simulink model "leon_chen_TDPBehaviourSim2"  (R2020b)
settings: Solver=FixedStepDiscrete  StartTime=0.0  StopTime=inf  RelTol=1e-3  EnableMultiTasking=on
values from neighbouring files (symbols this model uses):
  angThresh = pi/16    (= 0.196349540849)    [GameParameters.m]
  attackerKickSpeed = 0.3    [GameParameters.m]
  AwayFormation1 = [9.5 4 pi ... (first row only)    [FormationPoses.m]    (also in GameParameters.m)
  ballThresh = playerRadius + 0.03    (= 0.11)    [GameParameters.m]
  distThresh = 0.1    [GameParameters.m]
  fieldCenter = [mean(fieldLimitsX) mean(fieldLimitsY)]    [GameParameters.m]
  fieldLimitsX = [1 10]    [GameParameters.m]
  fieldLimitsY = [1 7]    [GameParameters.m]
  goalPosts = [1  2.7 2 ... (first row only)    [GameParameters.m]
  HomeFormation1 = [1.5 4 0 ... (first row only)    [FormationPoses.m]    (also in GameParameters.m)
  maxSpeed = 0.1    [GameParameters.m]
  maxTurnSpeed = 0.05    [GameParameters.m]
  playerRadius = 0.08    [GameParameters.m]
  robotDetectorAngle = 0    [GameParameters.m]
  robotDetectorFOV = 4.15    [GameParameters.m]
  robotDetectorMaxHits = 7    [GameParameters.m]
  robotDetectorOffset = [0 0]    [GameParameters.m]
  robotDetectorRange = 10    [GameParameters.m]
  sampleTime = 0.5    [GameParameters.m]
undefined symbols (not defined in the file or in its folder): DiscIntNeverNeededParam
libraries: mobileRoboticsLib x28, soccerRobotLib x16
(part 1 of 2)
settings Model: Creator=2683935i  LastModifiedBy=2692920R
settings SolverCC: AutoInsertRateTranBlk=on
settings DataIOCC: SaveOutput=off  SaveTime=off
settings OptimizationCC: DefaultParameterBehavior=Inlined  InlineInvariantSignals=on  EnhancedBackFolding=on  PassReuseOutputArgsAs=Individual arguments  StateBitsets=on  DataBitsets=on  ZeroExternalMemoryAtStartup=off  ZeroInternalMemoryAtStartup=off  NoFixptDivByZeroProtection=on  LifeSpan=1  OptimizeBlockOrder=speed  DifferentSizesBufferReuse=on  EfficientTunableParamExpr=on
settings DebuggingCC: MultiTaskRateTransMsg=warning  ParameterTunabilityLossMsg=error
settings HardwareCC: ProdBitPerPointer=32  ProdBitPerSizeT=32  ProdBitPerPtrDiffT=32  ProdLargestAtomicFloat=None  ProdIntDivRoundTo=Floor  ProdWordSize=32  ProdHWDeviceType=Generic->Custom
settings SFSimCC: MATLABDynamicMemAlloc=off
settings RTWCC: Description=Embedded Coder  SystemTargetFile=ert.tlc  TLCOptions=-p0  GenCodeOnly=on  TemplateMakefile=ert_default_tmf  GenerateReport=on  RTWVerbose=off  IncludeHyperlinkInReport=on  LaunchReport=on
settings CodeAppCC: ForceParamTrailComments=on  IgnoreCustomStorageClasses=off  OperatorAnnotations=on  SimulinkDataObjDesc=on  SFDataObjDesc=on  CustomSymbolStrGlobalVar=rt$N$M  CustomSymbolStrType=$N$M  CustomSymbolStrFcn=$N$M$F  CustomSymbolStrMacro=$N$M  InsertBlockDesc=on
settings ERTTargetCC: TargetLangStandard=C99 (ISO)  GenerateSampleERTMain=on  IncludeMdlTerminateFcn=off  SuppressErrorStatus=on  SupportAbsoluteTime=off  PurelyIntegerCode=on  SupportNonFinite=off  SupportComplex=off  InlinedParameterPlacement=NonHierarchical  RootIOFormat=Structure reference  ERTCustomFileTemplate=example_file_process.tlc

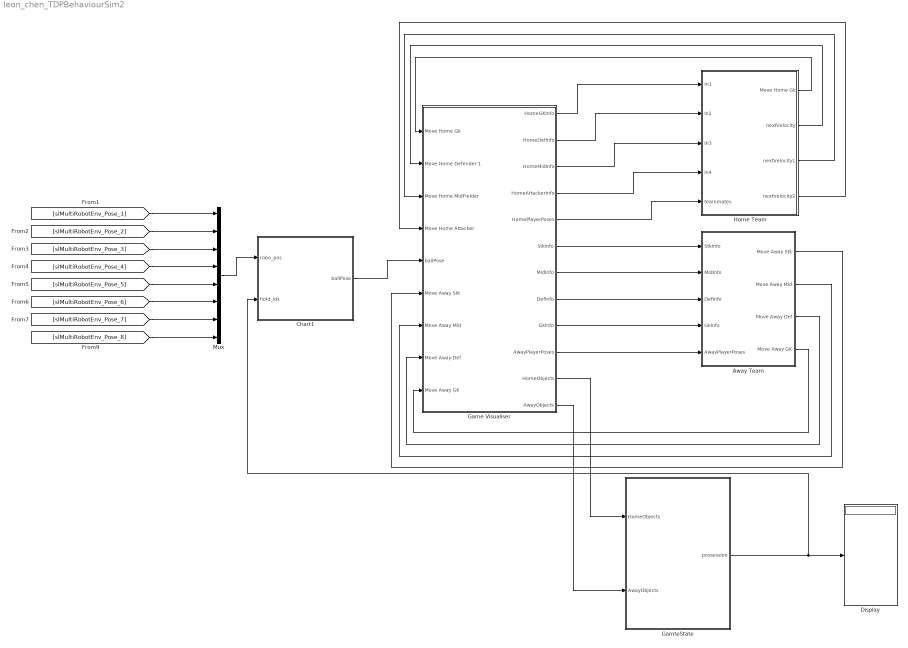
== system leon_chen_TDPBehaviourSim2 ==
  Away Team : Subsystem
  Chart1 : Stateflow chart  TreatAsAtomicUnit=on
  Display : Display
  Game Visualiser : Subsystem
  GamteState : Stateflow chart  TreatAsAtomicUnit=on
  Home Team : Subsystem
  Mux : Mux  Inputs=8
  wires:
  Away Team/2(Move Away Mid) -> Game Visualiser/7(Move Away Mid)
  Home Team/4(nextVelocity2) -> Game Visualiser/4(Move Home Attacker)
  Game Visualiser/5(HomePlayerPoses) -> Home Team/5(teammates)
  Home Team/1(Move Home Gk) -> Game Visualiser/1(Move Home Gk)
  Game Visualiser/1(HomeGKInfo) -> Home Team/1(In1)
  Home Team/2(nextVelocity) -> Game Visualiser/2(Move Home Defender 1)
  Away Team/4(Move Away GK) -> Game Visualiser/9(Move Away GK)
  Home Team/3(nextVelocity1) -> Game Visualiser/3(Move Home MidFielder)
  Game Visualiser/7(MidInfo) -> Away Team/2(MidInfo)
  Away Team/3(Move Away Def) -> Game Visualiser/8(Move Away Def)
  Chart1/1(ballPose) -> Game Visualiser/5(ballPose)
  Game Visualiser/9(GkInfo) -> Away Team/4(GkInfo)
  Game Visualiser/8(DefInfo) -> Away Team/3(DefInfo)
  Game Visualiser/6(StkInfo) -> Away Team/1(StkInfo)
  Game Visualiser/3(HomeMidInfo) -> Home Team/3(In3)
  Game Visualiser/4(HomeAttackerInfo) -> Home Team/4(In4)
  Game Visualiser/2(HomeDefInfo) -> Home Team/2(In2)
  Away Team/1(Move Away Stk) -> Game Visualiser/6(Move Away Stk)
  Game Visualiser/10(AwayPlayerPoses) -> Away Team/5(AwayPlayerPoses)
  GamteState/1(possession) -> Chart1/2(hold_idx), Display/1
  Game Visualiser/11(HomeObjects) -> GamteState/1(HomeObjects)
  Game Visualiser/12(AwayObjects) -> GamteState/2(AwayObjects)
  [slMultiRobotEnv_Pose_1] -> Mux/1
  [slMultiRobotEnv_Pose_2] -> Mux/2
  [slMultiRobotEnv_Pose_3] -> Mux/3
  [slMultiRobotEnv_Pose_4] -> Mux/4
  [slMultiRobotEnv_Pose_5] -> Mux/5
  [slMultiRobotEnv_Pose_6] -> Mux/6
  [slMultiRobotEnv_Pose_7] -> Mux/7
  [slMultiRobotEnv_Pose_8] -> Mux/8
  Mux/1 -> Chart1/1(robo_pos)

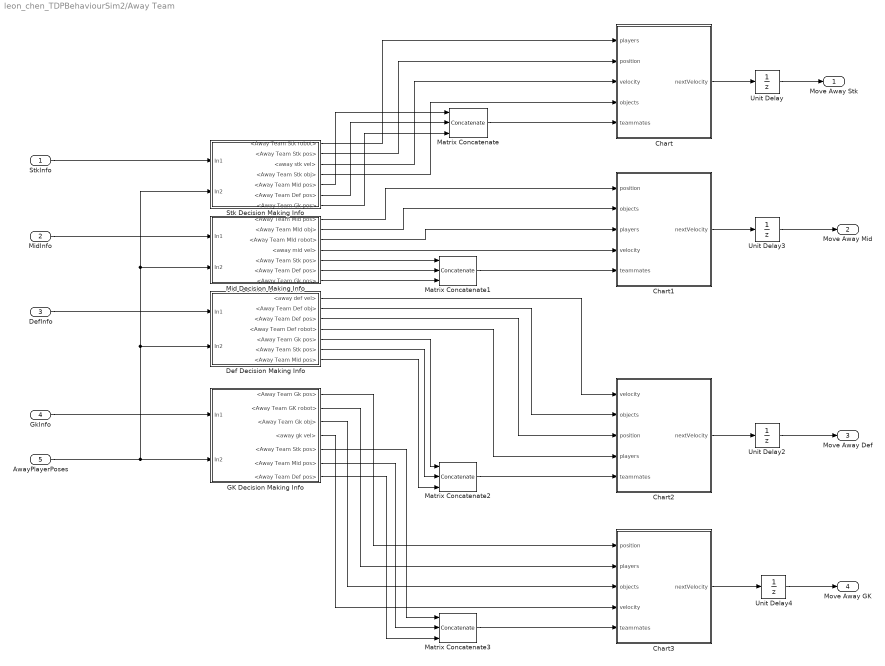
== system leon_chen_TDPBehaviourSim2/Away Team ==
  StkInfo : Inport
  MidInfo : Inport  Port=2
  DefInfo : Inport  Port=3
  GkInfo : Inport  Port=4
  AwayPlayerPoses : Inport  Port=5
  Chart : Stateflow chart  TreatAsAtomicUnit=on
      settings: PortSchema="{\"entries\":[{\"content\":{\"sides\":[{\"content\":{\"connectorIds\":[\"In3\",\"In1\",\"In2\",\"In5\",\"In4\"]},\"type\":\"ConnectorPlacement.EquallySpacedRectSide\",\"uuid\":\"cf890ef0-0ec1-422c-ab9c-1628c873ebf0\"},{\"content\":{\"connectorIds\":[\"Out1\"],\"side\":\"RIGHT\"},\"type\":\"ConnectorPlacement.EquallySpacedRectSide\",\"uuid\":\"0000e457-9393-40de-9950-8ff794b83dda\"},{\"content\":{\"connectorIds\":[],\"side\":\"TOP\"},\"type\":\"ConnectorPlacement.EquallySpacedRectSide\",\"uuid\":\"7dd8e30a-3952-4d7c-b255-0e0c48dee19a\"}]},\"type\":\"ConnectorPlacement.EquallySpacedConnector\",\"uuid\":\"e8168788-1535-41f0-a84f-110f92e839bd\"}],\"packageUris\":[\"http://schema.mathworks.com/mf0/Connector/R2020b\"],\"version\":\"1.0\"}"
  Chart1 : Stateflow chart  TreatAsAtomicUnit=on
      settings: PortSchema="{\"entries\":[{\"content\":{\"sides\":[{\"content\":{\"connectorIds\":[\"In1\",\"In5\",\"In3\",\"In2\",\"In4\"]},\"type\":\"ConnectorPlacement.EquallySpacedRectSide\",\"uuid\":\"cf890ef0-0ec1-422c-ab9c-1628c873ebf0\"},{\"content\":{\"connectorIds\":[\"Out1\"],\"side\":\"RIGHT\"},\"type\":\"ConnectorPlacement.EquallySpacedRectSide\",\"uuid\":\"0000e457-9393-40de-9950-8ff794b83dda\"},{\"content\":{\"connectorIds\":[],\"side\":\"TOP\"},\"type\":\"ConnectorPlacement.EquallySpacedRectSide\",\"uuid\":\"7dd8e30a-3952-4d7c-b255-0e0c48dee19a\"}]},\"type\":\"ConnectorPlacement.EquallySpacedConnector\",\"uuid\":\"e8168788-1535-41f0-a84f-110f92e839bd\"}],\"packageUris\":[\"http://schema.mathworks.com/mf0/Connector/R2020b\"],\"version\":\"1.0\"}"
  Chart2 : Stateflow chart  TreatAsAtomicUnit=on
      settings: PortSchema="{\"entries\":[{\"content\":{\"sides\":[{\"content\":{\"connectorIds\":[\"In2\",\"In5\",\"In1\",\"In3\",\"In4\"]},\"type\":\"ConnectorPlacement.EquallySpacedRectSide\",\"uuid\":\"cf890ef0-0ec1-422c-ab9c-1628c873ebf0\"},{\"content\":{\"connectorIds\":[\"Out1\"],\"side\":\"RIGHT\"},\"type\":\"ConnectorPlacement.EquallySpacedRectSide\",\"uuid\":\"0000e457-9393-40de-9950-8ff794b83dda\"},{\"content\":{\"connectorIds\":[],\"side\":\"TOP\"},\"type\":\"ConnectorPlacement.EquallySpacedRectSide\",\"uuid\":\"7dd8e30a-3952-4d7c-b255-0e0c48dee19a\"}]},\"type\":\"ConnectorPlacement.EquallySpacedConnector\",\"uuid\":\"e8168788-1535-41f0-a84f-110f92e839bd\"}],\"packageUris\":[\"http://schema.mathworks.com/mf0/Connector/R2020b\"],\"version\":\"1.0\"}"
  Chart3 : Stateflow chart  TreatAsAtomicUnit=on
      settings: PortSchema="{\"entries\":[{\"content\":{\"sides\":[{\"content\":{\"connectorIds\":[\"In1\",\"In3\",\"In5\",\"In2\",\"In4\"]},\"type\":\"ConnectorPlacement.EquallySpacedRectSide\",\"uuid\":\"cf890ef0-0ec1-422c-ab9c-1628c873ebf0\"},{\"content\":{\"connectorIds\":[\"Out1\"],\"side\":\"RIGHT\"},\"type\":\"ConnectorPlacement.EquallySpacedRectSide\",\"uuid\":\"0000e457-9393-40de-9950-8ff794b83dda\"},{\"content\":{\"connectorIds\":[],\"side\":\"TOP\"},\"type\":\"ConnectorPlacement.EquallySpacedRectSide\",\"uuid\":\"7dd8e30a-3952-4d7c-b255-0e0c48dee19a\"}]},\"type\":\"ConnectorPlacement.EquallySpacedConnector\",\"uuid\":\"e8168788-1535-41f0-a84f-110f92e839bd\"}],\"packageUris\":[\"http://schema.mathworks.com/mf0/Connector/R2020b\"],\"version\":\"1.0\"}"
  Def Decision Making Info : Subsystem
  GK Decision Making Info : Subsystem
  Matrix Concatenate{,1..3} (4 alike) : Concatenate  NumInputs=3  Mode=Multidimensional array
  Mid Decision Making Info : Subsystem
  Stk Decision Making Info : Subsystem
  Unit Delay{,2..4} (4 alike) : UnitDelay  SampleTime=-1  HasFrameUpgradeWarning=on
  Move Away Stk : Outport
  Move Away Mid : Outport  Port=2
  Move Away Def : Outport  Port=3
  Move Away GK : Outport  Port=4
  wires:
  Def Decision Making Info/7(<Away Team Mid pos>) -> Matrix Concatenate2/3
  Def Decision Making Info/6(<Away Team Stk pos>) -> Matrix Concatenate2/2
  AwayPlayerPoses/1 -> Stk Decision Making Info/2(In2), Mid Decision Making Info/2(In2), Def Decision Making Info/2(In2), GK Decision Making Info/2(In2)
  Def Decision Making Info/3(<Away Team Def pos>) -> Chart2/1(position)
  Matrix Concatenate3/1 -> Chart3/4(teammates)
  Unit Delay/1 -> Move Away Stk/1
  Stk Decision Making Info/6(<Away Team Def pos>) -> Matrix Concatenate/2
  Stk Decision Making Info/5(<Away Team Mid pos>) -> Matrix Concatenate/1
  Mid Decision Making Info/6(<Away Team Def pos>) -> Matrix Concatenate1/2
  Def Decision Making Info/1(<away def vel>) -> Chart2/2(velocity)
  Mid Decision Making Info/1(<Away Team Mid pos>) -> Chart1/1(position)
  Mid Decision Making Info/7(<Away Team Gk pos>) -> Matrix Concatenate1/3
  Mid Decision Making Info/4(<away mid vel>) -> Chart1/2(velocity)
  GK Decision Making Info/7(<Away Team Def pos>) -> Matrix Concatenate3/3
  GK Decision Making Info/2(<Away Team GK robot>) -> Chart3/3(players)
  GK Decision Making Info/1(<Away Team Gk pos>) -> Chart3/1(position)
  Matrix Concatenate/1 -> Chart/4(teammates)
  Stk Decision Making Info/4(<Away Team Stk obj>) -> Chart/5(objects)
  Chart1/1(nextVelocity) -> Unit Delay3/1
  Mid Decision Making Info/2(<Away Team MId obj>) -> Chart1/5(objects)
  Chart2/1(nextVelocity) -> Unit Delay2/1
  GkInfo/1 -> GK Decision Making Info/1(In1)
  Mid Decision Making Info/3(<Away Team MId robot>) -> Chart1/3(players)
  GK Decision Making Info/6(<Away Team Mid pos>) -> Matrix Concatenate3/2
  Chart/1(nextVelocity) -> Unit Delay/1
  Unit Delay4/1 -> Move Away GK/1
  Mid Decision Making Info/5(<Away Team Stk pos>) -> Matrix Concatenate1/1
  Def Decision Making Info/2(<Away Team Def obj>) -> Chart2/5(objects)
  Stk Decision Making Info/1(<Away Team Stk robot>) -> Chart/3(players)
  StkInfo/1 -> Stk Decision Making Info/1(In1)
  Def Decision Making Info/4(<Away Team Def robot>) -> Chart2/3(players)
  Chart3/1(nextVelocity) -> Unit Delay4/1
  Matrix Concatenate1/1 -> Chart1/4(teammates)
  GK Decision Making Info/3(<Away Team Gk obj>) -> Chart3/5(objects)
  Stk Decision Making Info/3(<away stk vel>) -> Chart/2(velocity)
  MidInfo/1 -> Mid Decision Making Info/1(In1)
  GK Decision Making Info/4(<away gk vel>) -> Chart3/2(velocity)
  Stk Decision Making Info/2(<Away Team Stk pos>) -> Chart/1(position)
  Matrix Concatenate2/1 -> Chart2/4(teammates)
  Stk Decision Making Info/7(<Away Team Gk pos>) -> Matrix Concatenate/3
  DefInfo/1 -> Def Decision Making Info/1(In1)
  Def Decision Making Info/5(<Away Team Gk pos>) -> Matrix Concatenate2/1
  Unit Delay2/1 -> Move Away Def/1
  GK Decision Making Info/5(<Away Team Stk pos>) -> Matrix Concatenate3/1
  Unit Delay3/1 -> Move Away Mid/1

== system leon_chen_TDPBehaviourSim2/Chart1/BallDynamics.InBounds.BallFree ==
  Action Port : ActionPort
      settings: CopyFcn=Stateflow.SLINSF.SimulinkMan.removeBlockPreDeleteFcn  PreDeleteFcn=Stateflow.SLINSF.SimulinkMan.unsafePredeleteFcn
  Gain : Gain  Gain=-0.25
  Position Integrator : DiscreteIntegrator  InitialCondition=fieldCenter  SampleTime=-1  StateName=ballPos  ICPrevOutput=DiscIntNeverNeededParam  ICPrevScaledInput=DiscIntNeverNeededParam
  Signal Specification : SignalSpecification  Dimensions=[1 2]
  Velocity Integrator : DiscreteIntegrator  InitialCondition=[0 0]  SampleTime=-1  StateName=ballVel  ICPrevOutput=DiscIntNeverNeededParam  ICPrevScaledInput=DiscIntNeverNeededParam
  ballPose : Outport  VectorParamsAs1DForOutWhenUnconnected=off
  wires:
  Gain/1 -> Velocity Integrator/1
  Velocity Integrator/1 -> Signal Specification/1
  Position Integrator/1 -> ballPose/1
  Signal Specification/1 -> Position Integrator/1, Gain/1

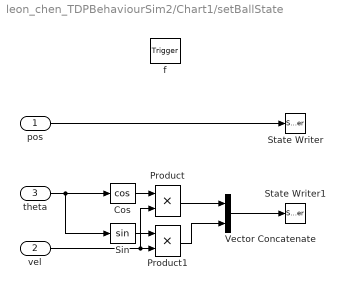
== system leon_chen_TDPBehaviourSim2/Chart1/setBallState ==
  pos : Inport  OutDataTypeStr=double  PortDimensions=[1 2]
  vel : Inport  Port=2  OutDataTypeStr=double  PortDimensions=1
  theta : Inport  Port=3  OutDataTypeStr=double  PortDimensions=1
  f : TriggerPort  TriggerType=function-call  VariantControl=(inherit)
      settings: CopyFcn=Stateflow.SLINSF.SimulinkMan.removeBlockPreDeleteFcn  PreDeleteFcn=Stateflow.SLINSF.SimulinkMan.unsafePredeleteFcn
  Cos : Trigonometry  Operator=cos
  Product : Product
  Product1 : Product
  Sin : Trigonometry
  State Writer : StateWriter  StateOwnerBlock=../../BallDynamics.InBounds.BallFree/Position Integrator  StateName=ballPos
  State Writer1 : StateWriter  StateOwnerBlock=../../BallDynamics.InBounds.BallFree/Velocity Integrator  StateName=ballVel
  Vector Concatenate : Concatenate  Mode=Multidimensional array  ConcatenateDimension=2
  wires:
  Vector Concatenate/1 -> State Writer1/1
  Product1/1 -> Vector Concatenate/2
  Product/1 -> Vector Concatenate/1
  theta/1 -> Cos/1, Sin/1
  Sin/1 -> Product1/1
  vel/1 -> Product1/2, Product/2
  Cos/1 -> Product/1
  pos/1 -> State Writer/1

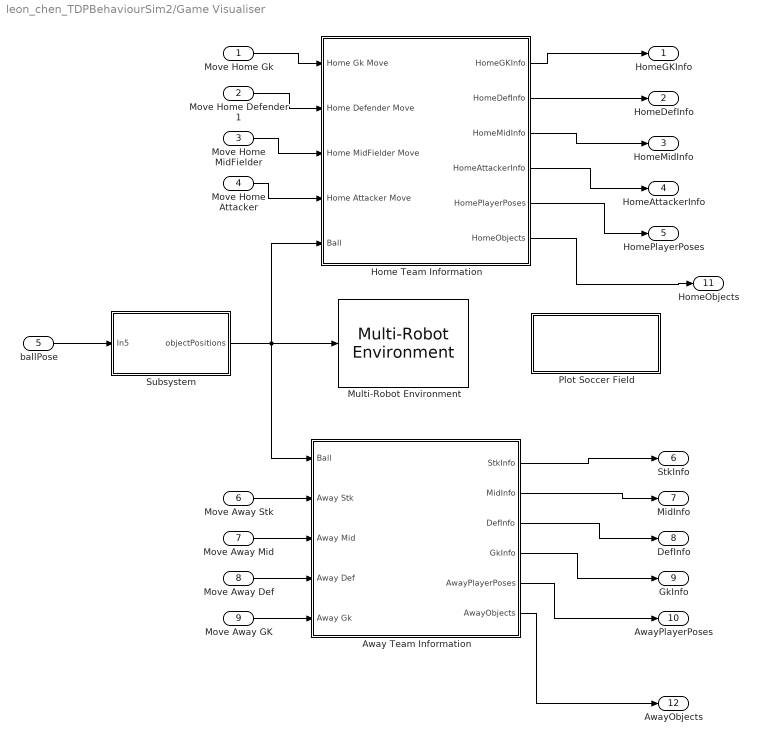
== system leon_chen_TDPBehaviourSim2/Game Visualiser ==
  Move Home Gk : Inport
  Move Home Defender 1 : Inport  Port=2
  Move Home MidFielder : Inport  Port=3
  Move Home Attacker : Inport  Port=4
  ballPose : Inport  Port=5
  Move Away Stk : Inport  Port=6
  Move Away Mid : Inport  Port=7
  Move Away Def : Inport  Port=8
  Move Away GK : Inport  Port=9
  Away Team Information : Subsystem
  Home Team Information : Subsystem
  Multi-Robot Environment : mobileRoboticsLib/Environments/Multi-Robot Environment  numRobots=numPlayers  mapName=map  showWaypoints=off  showObjects=on  objectColors=objColors  objectMarkers='o^^^^'  showRobotIds=on  plotSensorLines=off
      settings: SourceProductName=Mobile Robotics Simulation Toolbox
  Plot Soccer Field : MATLAB Function  TreatAsAtomicUnit=on
  Subsystem : Subsystem
  HomeGKInfo : Outport
  HomeDefInfo : Outport  Port=2
  HomeMidInfo : Outport  Port=3
  HomeAttackerInfo : Outport  Port=4
  HomePlayerPoses : Outport  Port=5
  StkInfo : Outport  Port=6
  MidInfo : Outport  Port=7
  DefInfo : Outport  Port=8
  GkInfo : Outport  Port=9
  AwayPlayerPoses : Outport  Port=10
  HomeObjects : Outport  Port=11
  AwayObjects : Outport  Port=12
  wires:
  Move Away Stk/1 -> Away Team Information/2(Away Stk)
  Move Home Defender 1/1 -> Home Team Information/2(Home Defender Move)
  Move Home MidFielder/1 -> Home Team Information/3(Home MidFielder Move)
  Move Away GK/1 -> Away Team Information/5("Away Gk ")
  Move Away Mid/1 -> Away Team Information/3(Away Mid)
  Move Away Def/1 -> Away Team Information/4(Away Def)
  Move Home Attacker/1 -> Home Team Information/4(Home Attacker Move)
  Move Home Gk/1 -> Home Team Information/1(Home Gk Move)
  Home Team Information/1(HomeGKInfo) -> HomeGKInfo/1
  Home Team Information/2(HomeDefInfo) -> HomeDefInfo/1
  Home Team Information/3(HomeMidInfo) -> HomeMidInfo/1
  Home Team Information/4(HomeAttackerInfo) -> HomeAttackerInfo/1
  Home Team Information/5(HomePlayerPoses) -> HomePlayerPoses/1
  Away Team Information/1(StkInfo) -> StkInfo/1
  Away Team Information/2(MidInfo) -> MidInfo/1
  Away Team Information/3(DefInfo) -> DefInfo/1
  Away Team Information/4(GkInfo) -> GkInfo/1
  Away Team Information/5(AwayPlayerPoses) -> AwayPlayerPoses/1
  Subsystem/1(objectPositions) -> Multi-Robot Environment/1, Away Team Information/1(Ball), Home Team Information/5(Ball)
  ballPose/1 -> Subsystem/1(In5)
  Home Team Information/6(HomeObjects) -> HomeObjects/1
  Away Team Information/6(AwayObjects) -> AwayObjects/1

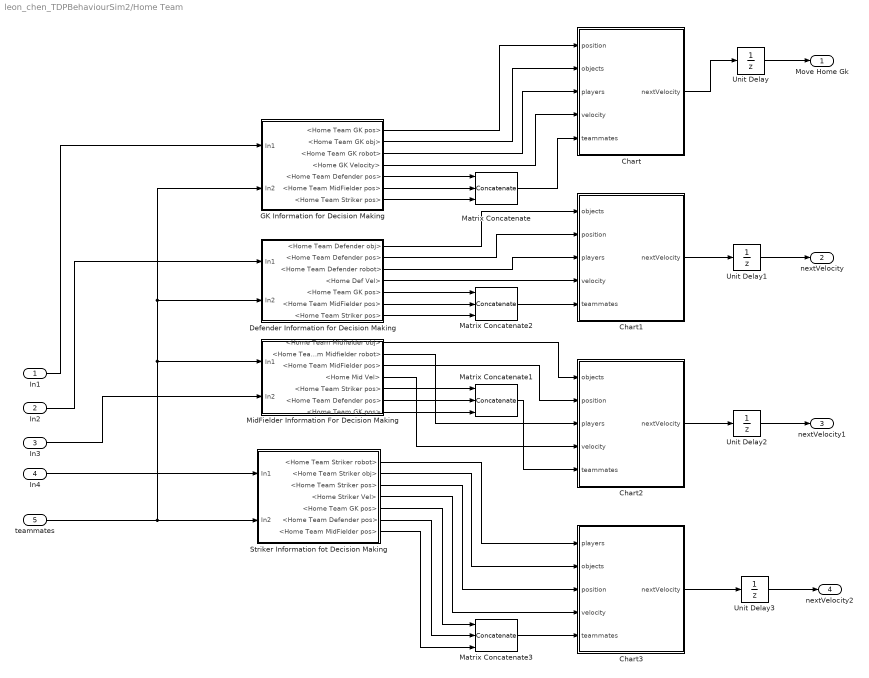
== system leon_chen_TDPBehaviourSim2/Home Team ==
  In1 : Inport
  In2 : Inport  Port=2
  In3 : Inport  Port=3
  In4 : Inport  Port=4
  teammates : Inport  Port=5
  Chart : Stateflow chart  TreatAsAtomicUnit=on
      settings: PortSchema="{\"entries\":[{\"content\":{\"sides\":[{\"content\":{\"connectorIds\":[\"In1\",\"In5\",\"In3\",\"In2\",\"In4\"]},\"type\":\"ConnectorPlacement.EquallySpacedRectSide\",\"uuid\":\"cf890ef0-0ec1-422c-ab9c-1628c873ebf0\"},{\"content\":{\"connectorIds\":[\"Out1\"],\"side\":\"RIGHT\"},\"type\":\"ConnectorPlacement.EquallySpacedRectSide\",\"uuid\":\"0000e457-9393-40de-9950-8ff794b83dda\"},{\"content\":{\"connectorIds\":[],\"side\":\"TOP\"},\"type\":\"ConnectorPlacement.EquallySpacedRectSide\",\"uuid\":\"7dd8e30a-3952-4d7c-b255-0e0c48dee19a\"}]},\"type\":\"ConnectorPlacement.EquallySpacedConnector\",\"uuid\":\"e8168788-1535-41f0-a84f-110f92e839bd\"}],\"packageUris\":[\"http://schema.mathworks.com/mf0/Connector/R2020b\"],\"version\":\"1.0\"}"
  Chart1 : Stateflow chart  TreatAsAtomicUnit=on
      settings: PortSchema="{\"entries\":[{\"content\":{\"sides\":[{\"content\":{\"connectorIds\":[\"In5\",\"In1\",\"In3\",\"In2\",\"In4\"]},\"type\":\"ConnectorPlacement.EquallySpacedRectSide\",\"uuid\":\"cf890ef0-0ec1-422c-ab9c-1628c873ebf0\"},{\"content\":{\"connectorIds\":[\"Out1\"],\"side\":\"RIGHT\"},\"type\":\"ConnectorPlacement.EquallySpacedRectSide\",\"uuid\":\"0000e457-9393-40de-9950-8ff794b83dda\"},{\"content\":{\"connectorIds\":[],\"side\":\"TOP\"},\"type\":\"ConnectorPlacement.EquallySpacedRectSide\",\"uuid\":\"7dd8e30a-3952-4d7c-b255-0e0c48dee19a\"}]},\"type\":\"ConnectorPlacement.EquallySpacedConnector\",\"uuid\":\"e8168788-1535-41f0-a84f-110f92e839bd\"}],\"packageUris\":[\"http://schema.mathworks.com/mf0/Connector/R2020b\"],\"version\":\"1.0\"}"
  Chart2 : Stateflow chart  TreatAsAtomicUnit=on
      settings: PortSchema="{\"entries\":[{\"content\":{\"sides\":[{\"content\":{\"connectorIds\":[\"In4\",\"In5\",\"In2\",\"In1\",\"In3\"]},\"type\":\"ConnectorPlacement.EquallySpacedRectSide\",\"uuid\":\"cf890ef0-0ec1-422c-ab9c-1628c873ebf0\"},{\"content\":{\"connectorIds\":[\"Out1\"],\"side\":\"RIGHT\"},\"type\":\"ConnectorPlacement.EquallySpacedRectSide\",\"uuid\":\"0000e457-9393-40de-9950-8ff794b83dda\"},{\"content\":{\"connectorIds\":[],\"side\":\"TOP\"},\"type\":\"ConnectorPlacement.EquallySpacedRectSide\",\"uuid\":\"7dd8e30a-3952-4d7c-b255-0e0c48dee19a\"}]},\"type\":\"ConnectorPlacement.EquallySpacedConnector\",\"uuid\":\"e8168788-1535-41f0-a84f-110f92e839bd\"}],\"packageUris\":[\"http://schema.mathworks.com/mf0/Connector/R2020b\"],\"version\":\"1.0\"}"
  Chart3 : Stateflow chart  TreatAsAtomicUnit=on
      settings: PortSchema="{\"entries\":[{\"content\":{\"sides\":[{\"content\":{\"connectorIds\":[\"In3\",\"In5\",\"In1\",\"In2\",\"In4\"]},\"type\":\"ConnectorPlacement.EquallySpacedRectSide\",\"uuid\":\"cf890ef0-0ec1-422c-ab9c-1628c873ebf0\"},{\"content\":{\"connectorIds\":[\"Out1\"],\"side\":\"RIGHT\"},\"type\":\"ConnectorPlacement.EquallySpacedRectSide\",\"uuid\":\"0000e457-9393-40de-9950-8ff794b83dda\"},{\"content\":{\"connectorIds\":[],\"side\":\"TOP\"},\"type\":\"ConnectorPlacement.EquallySpacedRectSide\",\"uuid\":\"7dd8e30a-3952-4d7c-b255-0e0c48dee19a\"}]},\"type\":\"ConnectorPlacement.EquallySpacedConnector\",\"uuid\":\"e8168788-1535-41f0-a84f-110f92e839bd\"}],\"packageUris\":[\"http://schema.mathworks.com/mf0/Connector/R2020b\"],\"version\":\"1.0\"}"
  "Defender Information for Decision Making " : Subsystem
  GK Information for Decision Making : Subsystem
  Matrix Concatenate : Concatenate  NumInputs=3  Mode=Multidimensional array  ConcatenateDimension=2
  Matrix Concatenate1 : Concatenate  NumInputs=3  Mode=Multidimensional array  ConcatenateDimension=2
  Matrix Concatenate2 : Concatenate  NumInputs=3  Mode=Multidimensional array  ConcatenateDimension=2
  Matrix Concatenate3 : Concatenate  NumInputs=3  Mode=Multidimensional array
  MidFielder Information For Decision Making : Subsystem
  Striker Information fot Decision Making : Subsystem
  Unit Delay{,1..3} (4 alike) : UnitDelay  SampleTime=-1  HasFrameUpgradeWarning=on
  Move Home Gk : Outport
  nextVelocity : Outport  Port=2
  nextVelocity1 : Outport  Port=3
  nextVelocity2 : Outport  Port=4
  wires:
  "Defender Information for Decision Making "/7(<Home Team Striker pos>) -> Matrix Concatenate2/3
  Matrix Concatenate3/1 -> Chart3/4(teammates)
  Matrix Concatenate1/1 -> Chart2/3(teammates)
  Striker Information fot Decision Making/7(<Home Team MidFielder pos>) -> Matrix Concatenate3/3
  Striker Information fot Decision Making/4(<Home Striker Vel>) -> Chart3/2(velocity)
  "Defender Information for Decision Making "/3(<Home Team Defender robot>) -> Chart1/3(players)
  GK Information for Decision Making/1(<Home Team GK pos>) -> Chart/1(position)
  In2/1 -> "Defender Information for Decision Making "/1(In1)
  GK Information for Decision Making/4(<Home GK Velocity>) -> Chart/2(velocity)
  teammates/1 -> GK Information for Decision Making/2(In2), "Defender Information for Decision Making "/2(In2), MidFielder Information For Decision Making/1(In1), Striker Information fot Decision Making/2(In2)
  Chart/1(nextVelocity) -> Unit Delay/1
  In4/1 -> Striker Information fot Decision Making/1(In1)
  "Defender Information for Decision Making "/6(<Home Team MidFielder pos>) -> Matrix Concatenate2/2
  GK Information for Decision Making/7(<Home Team Striker pos>) -> Matrix Concatenate/3
  In3/1 -> MidFielder Information For Decision Making/2(In2)
  MidFielder Information For Decision Making/3(<Home Team MidFielder pos>) -> Chart2/5(position)
  GK Information for Decision Making/3(<Home Team GK robot>) -> Chart/3(players)
  "Defender Information for Decision Making "/1(<Home Team Defender obj>) -> Chart1/5(objects)
  In1/1 -> GK Information for Decision Making/1(In1)
  "Defender Information for Decision Making "/4(<Home Def Vel>) -> Chart1/2(velocity)
  GK Information for Decision Making/5(<Home Team Defender pos>) -> Matrix Concatenate/1
  MidFielder Information For Decision Making/2(<Home Team Midfielder robot>) -> Chart2/2(players)
  GK Information for Decision Making/6(<Home Team MidFielder pos>) -> Matrix Concatenate/2
  Matrix Concatenate2/1 -> Chart1/4(teammates)
  Striker Information fot Decision Making/6(<Home Team Defender pos>) -> Matrix Concatenate3/2
  MidFielder Information For Decision Making/5(<Home Team Striker pos>) -> Matrix Concatenate1/1
  Striker Information fot Decision Making/3(<Home Team Striker pos>) -> Chart3/1(position)
  MidFielder Information For Decision Making/7(<Home Team GK pos>) -> Matrix Concatenate1/3
  GK Information for Decision Making/2(<Home Team GK obj>) -> Chart/5(objects)
  MidFielder Information For Decision Making/4(<Home Mid Vel>) -> Chart2/1(velocity)
  MidFielder Information For Decision Making/1(<Home Team Midfielder obj>) -> Chart2/4(objects)
  Striker Information fot Decision Making/2(<Home Team Striker obj>) -> Chart3/5(objects)
  Striker Information fot Decision Making/1(<Home Team Striker robot>) -> Chart3/3(players)
  Striker Information fot Decision Making/5(<Home Team GK pos>) -> Matrix Concatenate3/1
  Unit Delay/1 -> Move Home Gk/1
  MidFielder Information For Decision Making/6(<Home Team Defender pos>) -> Matrix Concatenate1/2
  "Defender Information for Decision Making "/2(<Home Team Defender pos>) -> Chart1/1(position)
  "Defender Information for Decision Making "/5(<Home Team GK pos>) -> Matrix Concatenate2/1
  Unit Delay3/1 -> nextVelocity2/1
  Chart3/1(nextVelocity) -> Unit Delay3/1
  Chart2/1(nextVelocity) -> Unit Delay2/1
  Unit Delay2/1 -> nextVelocity1/1
  Unit Delay1/1 -> nextVelocity/1
  Chart1/1(nextVelocity) -> Unit Delay1/1
  Matrix Concatenate/1 -> Chart/4(teammates)

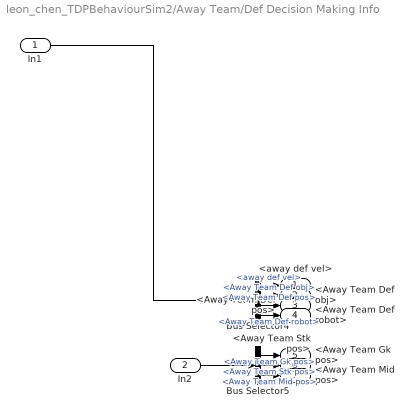
== system leon_chen_TDPBehaviourSim2/Away Team/Def Decision Making Info ==
  In1 : Inport
  In2 : Inport  Port=2
  Bus Selector4 : BusSelector  OutputSignals=away def vel,Away Team Def obj,Away Team Def pos,Away Team Def robot
  Bus Selector5 : BusSelector  OutputSignals=Away Team Gk pos,Away Team Stk pos,Away Team Mid pos
  <away def vel> : Outport
  <Away Team Def obj> : Outport  Port=2
  <Away Team Def pos> : Outport  Port=3
  <Away Team Def robot> : Outport  Port=4
  <Away Team Gk pos> : Outport  Port=5
  <Away Team Stk pos> : Outport  Port=6
  <Away Team Mid pos> : Outport  Port=7
  wires:
  Bus Selector5/2 -> <Away Team Stk pos>/1  "<Away Team Stk pos>"
  Bus Selector5/3 -> <Away Team Mid pos>/1  "<Away Team Mid pos>"
  Bus Selector4/2 -> <Away Team Def obj>/1  "<Away Team Def obj>"
  Bus Selector4/3 -> <Away Team Def pos>/1  "<Away Team Def pos>"
  Bus Selector4/1 -> <away def vel>/1  "<away def vel>"
  In2/1 -> Bus Selector5/1
  In1/1 -> Bus Selector4/1
  Bus Selector4/4 -> <Away Team Def robot>/1  "<Away Team Def robot>"
  Bus Selector5/1 -> <Away Team Gk pos>/1  "<Away Team Gk pos>"

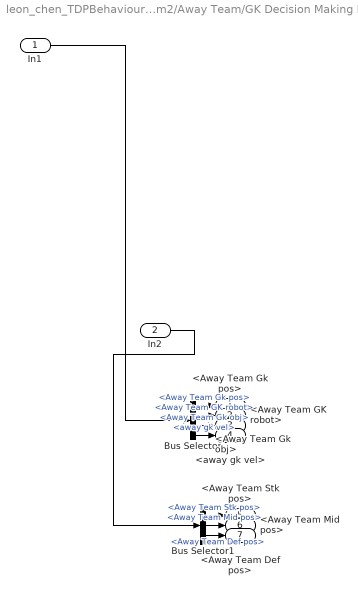
== system leon_chen_TDPBehaviourSim2/Away Team/GK Decision Making Info ==
  In1 : Inport
  In2 : Inport  Port=2
  Bus Selector : BusSelector  OutputSignals=Away Team Gk pos,Away Team GK robot,Away Team Gk obj,away gk vel
  Bus Selector1 : BusSelector  OutputSignals=Away Team Stk pos,Away Team Mid pos,Away Team Def pos
  <Away Team Gk pos> : Outport
  <Away Team GK robot> : Outport  Port=2
  <Away Team Gk obj> : Outport  Port=3
  <away gk vel> : Outport  Port=4
  <Away Team Stk pos> : Outport  Port=5
  <Away Team Mid pos> : Outport  Port=6
  <Away Team Def pos> : Outport  Port=7
  wires:
  In2/1 -> Bus Selector1/1
  Bus Selector/2 -> <Away Team GK robot>/1  "<Away Team GK robot>"
  Bus Selector/3 -> <Away Team Gk obj>/1  "<Away Team Gk obj>"
  In1/1 -> Bus Selector/1
  Bus Selector1/3 -> <Away Team Def pos>/1  "<Away Team Def pos>"
  Bus Selector/1 -> <Away Team Gk pos>/1  "<Away Team Gk pos>"
  Bus Selector1/1 -> <Away Team Stk pos>/1  "<Away Team Stk pos>"
  Bus Selector/4 -> <away gk vel>/1  "<away gk vel>"
  Bus Selector1/2 -> <Away Team Mid pos>/1  "<Away Team Mid pos>"

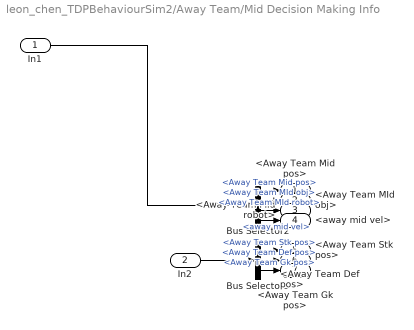
== system leon_chen_TDPBehaviourSim2/Away Team/Mid Decision Making Info ==
  In1 : Inport
  In2 : Inport  Port=2
  Bus Selector2 : BusSelector  OutputSignals=Away Team Mid pos,Away Team MId obj,Away Team MId robot,away mid vel
  Bus Selector3 : BusSelector  OutputSignals=Away Team Stk pos,Away Team Def pos,Away Team Gk pos
  <Away Team Mid pos> : Outport
  <Away Team MId obj> : Outport  Port=2
  <Away Team MId robot> : Outport  Port=3
  <away mid vel> : Outport  Port=4
  <Away Team Stk pos> : Outport  Port=5
  <Away Team Def pos> : Outport  Port=6
  <Away Team Gk pos> : Outport  Port=7
  wires:
  Bus Selector2/2 -> <Away Team MId obj>/1  "<Away Team MId obj>"
  Bus Selector3/1 -> <Away Team Stk pos>/1  "<Away Team Stk pos>"
  Bus Selector2/3 -> <Away Team MId robot>/1  "<Away Team MId robot>"
  In1/1 -> Bus Selector2/1
  Bus Selector3/2 -> <Away Team Def pos>/1  "<Away Team Def pos>"
  Bus Selector3/3 -> <Away Team Gk pos>/1  "<Away Team Gk pos>"
  In2/1 -> Bus Selector3/1
  Bus Selector2/1 -> <Away Team Mid pos>/1  "<Away Team Mid pos>"
  Bus Selector2/4 -> <away mid vel>/1  "<away mid vel>"

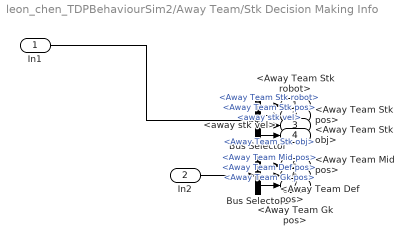
== system leon_chen_TDPBehaviourSim2/Away Team/Stk Decision Making Info ==
  In1 : Inport
  In2 : Inport  Port=2
  Bus Selector : BusSelector  OutputSignals=Away Team Stk robot,Away Team Stk pos,away stk vel,Away Team Stk obj
  Bus Selector1 : BusSelector  OutputSignals=Away Team Mid pos,Away Team Def pos,Away Team Gk pos
  <Away Team Stk robot> : Outport
  <Away Team Stk pos> : Outport  Port=2
  <away stk vel> : Outport  Port=3
  <Away Team Stk obj> : Outport  Port=4
  <Away Team Mid pos> : Outport  Port=5
  <Away Team Def pos> : Outport  Port=6
  <Away Team Gk pos> : Outport  Port=7
  wires:
  In2/1 -> Bus Selector1/1
  Bus Selector/3 -> <away stk vel>/1  "<away stk vel>"
  Bus Selector1/2 -> <Away Team Def pos>/1  "<Away Team Def pos>"
  Bus Selector/4 -> <Away Team Stk obj>/1  "<Away Team Stk obj>"
  Bus Selector1/3 -> <Away Team Gk pos>/1  "<Away Team Gk pos>"
  Bus Selector/1 -> <Away Team Stk robot>/1  "<Away Team Stk robot>"
  Bus Selector1/1 -> <Away Team Mid pos>/1  "<Away Team Mid pos>"
  Bus Selector/2 -> <Away Team Stk pos>/1  "<Away Team Stk pos>"
  In1/1 -> Bus Selector/1

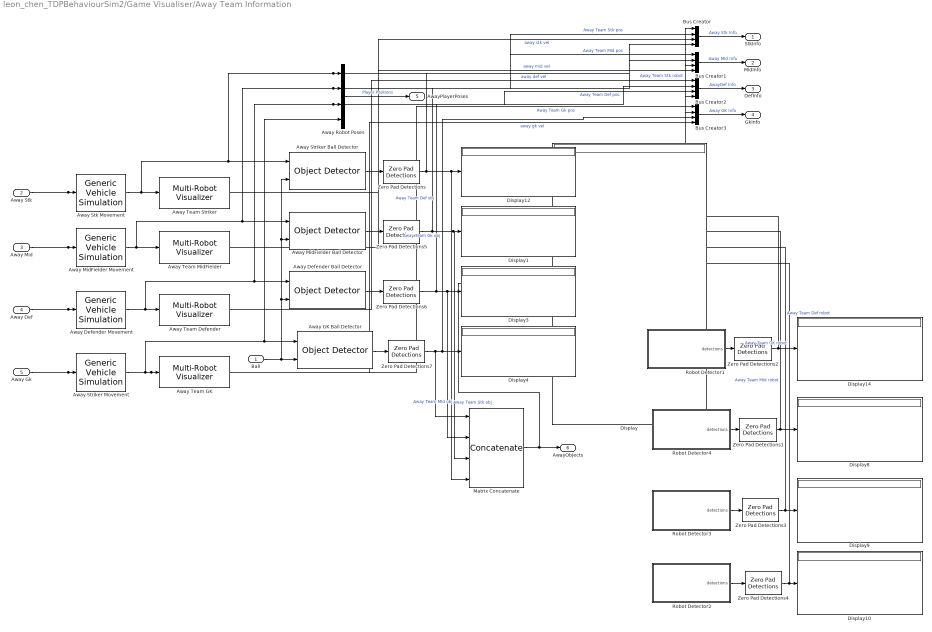
== system leon_chen_TDPBehaviourSim2/Game Visualiser/Away Team Information ==
  Ball : Inport
  Away Stk : Inport  Port=2
  Away Mid : Inport  Port=3
  Away Def : Inport  Port=4
  "Away Gk " : Inport  Port=5
  Away Defender Ball Detector : mobileRoboticsLib/Environments/Object Detector  mapName=map  sensorOffset=objDetectorOffset  sensorAngle=objDetectorAngle  fieldOfView=objDetectorFOV  maxRange=objDetectorRange  maxDetections=objDetectorMaxHits  sampleTime=sampleTime
      settings: SourceProductName=Mobile Robotics Simulation Toolbox
  Away Defender Movement : mobileRoboticsLib/Utilities/Generic Vehicle Simulation  initX=AwayFormation1(2,1)  initY=AwayFormation1(2,2)  initAngle=AwayFormation1(2,3)  Ts=0.05
      settings: SourceProductName=Mobile Robotics Simulation Toolbox
  Away GK Ball Detector : mobileRoboticsLib/Environments/Object Detector  mapName=map  sensorOffset=objDetectorOffset  sensorAngle=objDetectorAngle  fieldOfView=objDetectorFOV  maxRange=objDetectorRange  maxDetections=objDetectorMaxHits  sampleTime=sampleTime
      settings: SourceProductName=Mobile Robotics Simulation Toolbox
  Away MidFielder Ball Detector : mobileRoboticsLib/Environments/Object Detector  mapName=map  sensorOffset=objDetectorOffset  sensorAngle=objDetectorAngle  fieldOfView=objDetectorFOV  maxRange=objDetectorRange  maxDetections=objDetectorMaxHits  sampleTime=sampleTime
      settings: SourceProductName=Mobile Robotics Simulation Toolbox
  Away MidFielder Movement : mobileRoboticsLib/Utilities/Generic Vehicle Simulation  initX=AwayFormation1(3,1)  initY=AwayFormation1(3,2)  initAngle=AwayFormation1(3,3)  Ts=0.05
      settings: SourceProductName=Mobile Robotics Simulation Toolbox
  Away Robot Poses : BusCreator  Inputs=4
  Away Stk Movement : mobileRoboticsLib/Utilities/Generic Vehicle Simulation  initX=AwayFormation1(4,1)  initY=AwayFormation1(4,2)  initAngle=AwayFormation1(4,3)  Ts=0.05
      settings: SourceProductName=Mobile Robotics Simulation Toolbox
  Away Striker Ball Detector : mobileRoboticsLib/Environments/Object Detector  mapName=map  sensorOffset=objDetectorOffset  sensorAngle=objDetectorAngle  fieldOfView=objDetectorFOV  maxRange=objDetectorRange  maxDetections=objDetectorMaxHits  sampleTime=sampleTime
      settings: SourceProductName=Mobile Robotics Simulation Toolbox
  Away Striker Movement : mobileRoboticsLib/Utilities/Generic Vehicle Simulation  initX=AwayFormation1(1,1)  initY=AwayFormation1(1,2)  initAngle=AwayFormation1(1,3)  Ts=0.05
      settings: SourceProductName=Mobile Robotics Simulation Toolbox
  Away Team Defender : mobileRoboticsLib/Environments/Multi-Robot Visualizer  idx=7  radius=playerRadius  robotColor=awayTeamColor  showTraj=on  hasLidar=off  sensorOffset=[0,0]  scanAngles=[-pi/4 0 pi/4]  maxNumScans=0  hasObjDetector=on  objDetectorOffset=objDetectorOffset  objDetectorAngle=objDetectorAngle  objDetectorFOV=objDetectorFOV  objDetectorMaxRange=objDetectorRange  hasRobotDetector=on  robotDetectorOffset=robotDetectorOffset  robotDetectorAngle=robotDetectorAngle  robotDetectorFOV=robotDetectorFOV  robotDetectorMaxRange=robotDetectorMaxHits  robotDetectorNumDetections=0
      settings: SourceProductName=Mobile Robotics Simulation Toolbox
  Away Team GK : mobileRoboticsLib/Environments/Multi-Robot Visualizer  idx=8  radius=playerRadius  robotColor=awayGKColor  showTraj=on  hasLidar=off  sensorOffset=[0,0]  scanAngles=[-pi/4 0 pi/4]  maxNumScans=0  hasObjDetector=on  objDetectorOffset=objDetectorOffset  objDetectorAngle=objDetectorAngle  objDetectorFOV=objDetectorFOV  objDetectorMaxRange=objDetectorRange  hasRobotDetector=on  robotDetectorOffset=robotDetectorOffset  robotDetectorAngle=robotDetectorAngle  robotDetectorFOV=robotDetectorFOV  robotDetectorMaxRange=robotDetectorMaxHits  robotDetectorNumDetections=0
      settings: SourceProductName=Mobile Robotics Simulation Toolbox
  Away Team MidFielder : mobileRoboticsLib/Environments/Multi-Robot Visualizer  idx=6  radius=playerRadius  robotColor=awayTeamColor  showTraj=on  hasLidar=off  sensorOffset=[0,0]  scanAngles=[-pi/4 0 pi/4]  maxNumScans=0  hasObjDetector=on  objDetectorOffset=objDetectorOffset  objDetectorAngle=objDetectorAngle  objDetectorFOV=objDetectorFOV  objDetectorMaxRange=objDetectorRange  hasRobotDetector=on  robotDetectorOffset=robotDetectorOffset  robotDetectorAngle=robotDetectorAngle  robotDetectorFOV=robotDetectorFOV  robotDetectorMaxRange=robotDetectorMaxHits  robotDetectorNumDetections=0
      settings: SourceProductName=Mobile Robotics Simulation Toolbox
  Away Team Striker : mobileRoboticsLib/Environments/Multi-Robot Visualizer  idx=5  radius=playerRadius  robotColor=awayTeamColor  showTraj=on  hasLidar=off  sensorOffset=[0,0]  scanAngles=[-pi/4 0 pi/4]  maxNumScans=0  hasObjDetector=on  objDetectorOffset=objDetectorOffset  objDetectorAngle=objDetectorAngle  objDetectorFOV=objDetectorFOV  objDetectorMaxRange=objDetectorRange  hasRobotDetector=on  robotDetectorOffset=robotDetectorOffset  robotDetectorAngle=robotDetectorAngle  robotDetectorFOV=robotDetectorFOV  robotDetectorMaxRange=robotDetectorMaxHits  robotDetectorNumDetections=0
      settings: SourceProductName=Mobile Robotics Simulation Toolbox
  Bus Creator{,1..3} (4 alike) : BusCreator  Inputs=4
  Display{,1,3..4,8..10,12,14} (9 alike) : Display
  Matrix Concatenate : Concatenate  NumInputs=4  Mode=Multidimensional array
  Robot Detector1 : Subsystem  AncestorBlock=mobileRoboticsLib/Environments/Robot Detector  mask(Robot Detector){mapName=map, robotIdx=5, sensorOffset=robotDetectorOffset, sensorAngle=robotDetectorAngle, sensorFOV=robotDetectorFOV, maxRange=robotDetectorRange, maxDetections=robotDetectorMaxHits, sampleTime=sampleTime}
      mask prompts: mapName "Map Name"; robotIdx "Robot Index"; sensorOffset "Sensor offset (x,y) [m]"; sensorAngle "Sensor angle [rad]"; sensorFOV "Sensor field of view [rad]"; maxRange "Maximum range [rad]"; maxDetections "Maximum number of detections"; sampleTime "Sample Time"
      mask help: Robot Detector Simulator
      mask init:
      | % Find number of robots 
      | mrEnvBlks = find_system(bdroot,'FollowLinks','on','LookUnderMasks','on','MaskType','Multi-Robot Environment');
      | mrEnvBlk = mrEnvBlks{1};
      | if isempty(mrEnvBlk)
      |     error('No Multi-Robot Environment found in model.')
      | end
      | numRobots = evalin('base',get_param(mrEnvBlk,'numRobots'));
      | 
      | % Configure pose tags
      | poseSub = [gcb '/Poses'];
      | poseBlocks = find_system(poseSub,'FollowLinks','on','LookUnderMasks','on','BlockType','From');
      | for idx = 1:numel(poseBlocks)
      |     lh = get_param(poseBlocks{idx},'LineHandles');
      |     delete_line(lh.Outport);
      | end
      | delete_block(poseBlocks);
      | vecBlock = [poseSub '/Vector Concatenate'];
      | set_param(vecBlock,'NumInputs',num2str(numRobots));
      | for idx = 1:numRobots
      |     blkName = [poseSub '/From' num2str(idx)];
      |     blkPos = [0 30 200 50] + (idx-1)*[0 30 0 30];
      |     add_block('simulink/Signal Routing/From',blkName);
      |     set_param(blkName,'GotoTag',['slMultiRobotEnv_Pose_' num2str(idx)]);
      |     set_param(blkName,'Position',blkPos);
      |     add_line(poseSub,['From' num2str(idx) '/1'],['Vector Concatenate/' num2str(idx)]);
      | end
      mask Help: web('matlab: edit mrsDocRobotDetector')
      mask Callback mapName:
      | % Update the map in the Robot Detector system object inside the mask
      | mapName = get_param(gcb,'mapName');
      | blkName = [gcb '/Robot Detector'];
      | set_param(blkName,'mapName',mapName);
      mask Display:
      | idx = get_param(gcb,'robotIdx');
      | fprintf(['Robot ' idx '\n Detector'])
  Robot Detector2 : Subsystem  AncestorBlock=mobileRoboticsLib/Environments/Robot Detector  mask(Robot Detector){mapName=map, robotIdx=8, sensorOffset=robotDetectorOffset, sensorAngle=robotDetectorAngle, sensorFOV=robotDetectorFOV, maxRange=robotDetectorRange, maxDetections=robotDetectorMaxHits, sampleTime=sampleTime}
      mask prompts: mapName "Map Name"; robotIdx "Robot Index"; sensorOffset "Sensor offset (x,y) [m]"; sensorAngle "Sensor angle [rad]"; sensorFOV "Sensor field of view [rad]"; maxRange "Maximum range [rad]"; maxDetections "Maximum number of detections"; sampleTime "Sample Time"
      mask help: Robot Detector Simulator
      mask init: same as leon_chen_TDPBehaviourSim2/Game Visualiser/Away Team Information/Robot Detector1
      mask Help: web('matlab: edit mrsDocRobotDetector')
      mask Callback mapName:
      | % Update the map in the Robot Detector system object inside the mask
      | mapName = get_param(gcb,'mapName');
      | blkName = [gcb '/Robot Detector'];
      | set_param(blkName,'mapName',mapName);
      mask Display:
      | idx = get_param(gcb,'robotIdx');
      | fprintf(['Robot ' idx '\n Detector'])
  Robot Detector3 : Subsystem  AncestorBlock=mobileRoboticsLib/Environments/Robot Detector  mask(Robot Detector){mapName=map, robotIdx=7, sensorOffset=robotDetectorOffset, sensorAngle=robotDetectorAngle, sensorFOV=robotDetectorFOV, maxRange=robotDetectorRange, maxDetections=robotDetectorMaxHits, sampleTime=sampleTime}
      mask prompts: mapName "Map Name"; robotIdx "Robot Index"; sensorOffset "Sensor offset (x,y) [m]"; sensorAngle "Sensor angle [rad]"; sensorFOV "Sensor field of view [rad]"; maxRange "Maximum range [rad]"; maxDetections "Maximum number of detections"; sampleTime "Sample Time"
      mask help: Robot Detector Simulator
      mask init: same as leon_chen_TDPBehaviourSim2/Game Visualiser/Away Team Information/Robot Detector1
      mask Help: web('matlab: edit mrsDocRobotDetector')
      mask Callback mapName:
      | % Update the map in the Robot Detector system object inside the mask
      | mapName = get_param(gcb,'mapName');
      | blkName = [gcb '/Robot Detector'];
      | set_param(blkName,'mapName',mapName);
      mask Display:
      | idx = get_param(gcb,'robotIdx');
      | fprintf(['Robot ' idx '\n Detector'])
  Robot Detector4 : Subsystem  AncestorBlock=mobileRoboticsLib/Environments/Robot Detector  mask(Robot Detector){mapName=map, robotIdx=6, sensorOffset=robotDetectorOffset, sensorAngle=robotDetectorAngle, sensorFOV=robotDetectorFOV, maxRange=robotDetectorRange, maxDetections=robotDetectorMaxHits, sampleTime=sampleTime}
      mask prompts: mapName "Map Name"; robotIdx "Robot Index"; sensorOffset "Sensor offset (x,y) [m]"; sensorAngle "Sensor angle [rad]"; sensorFOV "Sensor field of view [rad]"; maxRange "Maximum range [rad]"; maxDetections "Maximum number of detections"; sampleTime "Sample Time"
      mask help: Robot Detector Simulator
      mask init: same as leon_chen_TDPBehaviourSim2/Game Visualiser/Away Team Information/Robot Detector1
      mask Help: web('matlab: edit mrsDocRobotDetector')
      mask Callback mapName:
      | % Update the map in the Robot Detector system object inside the mask
      | mapName = get_param(gcb,'mapName');
      | blkName = [gcb '/Robot Detector'];
      | set_param(blkName,'mapName',mapName);
      mask Display:
      | idx = get_param(gcb,'robotIdx');
      | fprintf(['Robot ' idx '\n Detector'])
  Zero Pad Detections{,5..7} (4 alike) : soccerRobotLib/Soccer Robot Simulator/Zero Pad Detections  maxHits=objDetectorMaxHits
  Zero Pad Detections{1..4} (4 alike) : soccerRobotLib/Soccer Robot Simulator/Zero Pad Detections  maxHits=robotDetectorMaxHits
  StkInfo : Outport
  MidInfo : Outport  Port=2
  DefInfo : Outport  Port=3
  GkInfo : Outport  Port=4
  AwayPlayerPoses : Outport  Port=5
  AwayObjects : Outport  Port=6
  wires:
  "Away Gk "/1 -> Bus Creator3/4, Away Striker Movement/1  "away gk vel"
  Away Def/1 -> Away Defender Movement/1, Bus Creator2/1  "away def vel"
  Ball/1 -> Away Striker Ball Detector/2, Away MidFielder Ball Detector/2, Away Defender Ball Detector/2, Away GK Ball Detector/2
  Away Striker Ball Detector/1 -> Zero Pad Detections/1
  Away Defender Ball Detector/1 -> Zero Pad Detections6/1
  Away MidFielder Ball Detector/1 -> Zero Pad Detections5/1
  Away GK Ball Detector/1 -> Zero Pad Detections7/1
  Zero Pad Detections/1 -> Matrix Concatenate/4, Display12/1, Bus Creator/4  "Away Team Stk obj"
  Zero Pad Detections5/1 -> Bus Creator1/2, Matrix Concatenate/3, Display1/1  "Away Team MId obj"
  Zero Pad Detections6/1 -> Bus Creator2/2, Matrix Concatenate/2, Display3/1  "Away Team Def obj"
  Zero Pad Detections7/1 -> Matrix Concatenate/1, Display4/1, Bus Creator3/3  "Away Team Gk obj"
  Away Striker Movement/1 -> Bus Creator3/1, Away Team GK/1, Away Robot Poses/4, Away GK Ball Detector/1  "Away Team Gk pos"
  Away MidFielder Movement/1 -> Away Team MidFielder/1, Away MidFielder Ball Detector/1, Bus Creator1/1, Away Robot Poses/2  "Away Team Mid pos"
  Away Stk Movement/1 -> Bus Creator/2, Away Robot Poses/1, Away Striker Ball Detector/1, Away Team Striker/1  "Away Team Stk pos"
  Away Defender Movement/1 -> Away Defender Ball Detector/1, Away Robot Poses/3, Bus Creator2/3, Away Team Defender/1  "Away Team Def pos"
  Zero Pad Detections1/1 -> Bus Creator1/3, Display8/1  "Away Team MId robot"
  Zero Pad Detections3/1 -> Display9/1, Bus Creator2/4  "Away Team Def robot"
  Robot Detector1/1(detections) -> Zero Pad Detections2/1
  Robot Detector4/1(detections) -> Zero Pad Detections1/1
  Robot Detector3/1(detections) -> Zero Pad Detections3/1
  Robot Detector2/1(detections) -> Zero Pad Detections4/1
  Zero Pad Detections4/1 -> Display10/1, Bus Creator3/2  "Away Team GK robot"
  Zero Pad Detections2/1 -> Bus Creator/1, Display14/1  "Away Team Stk robot"
  Away Stk/1 -> Bus Creator/3, Away Stk Movement/1  "away stk vel"
  Away Mid/1 -> Bus Creator1/4, Away MidFielder Movement/1  "away mid vel"
  Bus Creator/1 -> StkInfo/1  "Away Stk Info"
  Bus Creator1/1 -> MidInfo/1  "Away MId Info"
  Bus Creator2/1 -> DefInfo/1  "AwayDef Info"
  Bus Creator3/1 -> GkInfo/1  "Away GK Info"
  Away Robot Poses/1 -> AwayPlayerPoses/1  "Player Positions"
  Matrix Concatenate/1 -> Display/1, AwayObjects/1
